simulink model "hexapod"  (R2022a)
settings: Solver=ode2  StartTime=0.0  StopTime=10.0  FixedStep=1e-4  RelTol=1e-3  AbsTol=1e-3  EnableMultiTasking=on
values from neighbouring files (symbols this model uses):
  N = 2    [gen_singleGait.m]
  s = t/T    [gait_mv_backward.m]    (also in gait_mv_forward.m; gait_mv_left.m; gait_mv_right.m; gait_rot_clockwise.m)
undefined symbols (not defined in the file or in its folder): X, Y, Z
libraries: sm_lib x90, nesl_utility x19, Contact_Forces_Lib x6, simulink x1
(part 2 of 4)

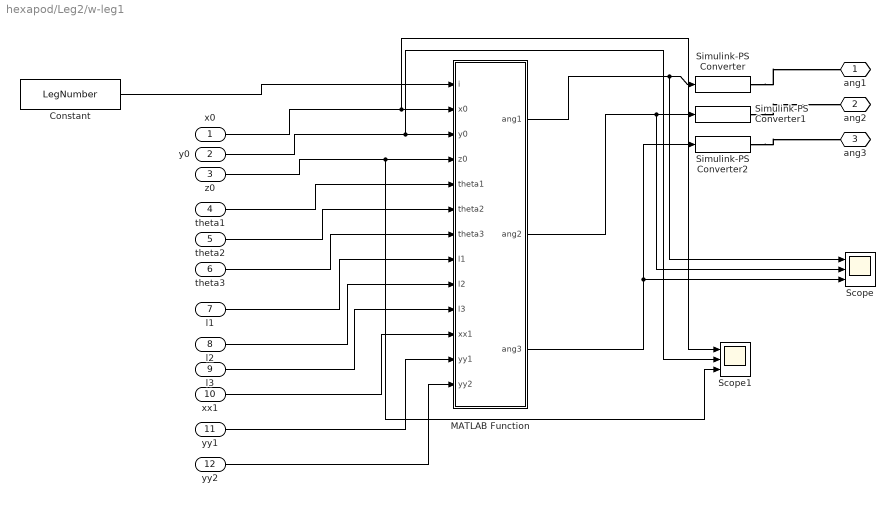
== system hexapod/Leg2/w-leg1 ==
  x0 : Inport
  y0 : Inport  Port=2
  z0 : Inport  Port=3
  theta1 : Inport  Port=4
  theta2 : Inport  Port=5
  theta3 : Inport  Port=6
  l1 : Inport  Port=7
  l2 : Inport  Port=8
  l3 : Inport  Port=9
  xx1 : Inport  Port=10
  yy1 : Inport  Port=11
  yy2 : Inport  Port=12
  Constant : Constant  Value=LegNumber
  MATLAB Function : MATLAB Function  TreatAsAtomicUnit=on
  Scope : Scope  NumInputPorts=3
  Scope1 : Scope  NumInputPorts=3
  Simulink-PS Converter : nesl_utility/Simulink-PS Converter  PhysicalDomain=network_engine_domain  SubClassName=ps_input  LeftPortType=input  RightPortType=output  PseudoPeriodic=off  Frequencies=[]  NoiseDistribution=none  NoiseParameters=[]  Unit=1  AffineConversion=off  FilteringAndDerivatives=filter  SimscapeFilterOrder=2  InputFilterTimeConstant=0.001  UdotUserProvided=0
      settings: SourceProductBaseCode=SS,PW,VE
  Simulink-PS Converter1 : nesl_utility/Simulink-PS Converter  PhysicalDomain=network_engine_domain  SubClassName=ps_input  LeftPortType=input  RightPortType=output  PseudoPeriodic=off  Frequencies=[]  NoiseDistribution=none  NoiseParameters=[]  Unit=1  AffineConversion=off  FilteringAndDerivatives=filter  SimscapeFilterOrder=2  InputFilterTimeConstant=0.001  UdotUserProvided=0
      settings: SourceProductBaseCode=SS,PW,VE
  Simulink-PS Converter2 : nesl_utility/Simulink-PS Converter  PhysicalDomain=network_engine_domain  SubClassName=ps_input  LeftPortType=input  RightPortType=output  PseudoPeriodic=off  Frequencies=[]  NoiseDistribution=none  NoiseParameters=[]  Unit=1  AffineConversion=off  FilteringAndDerivatives=filter  SimscapeFilterOrder=2  InputFilterTimeConstant=0.001  UdotUserProvided=0
      settings: SourceProductBaseCode=SS,PW,VE
  ang1 : PMIOPort  Side=Right
  ang2 : PMIOPort  Port=2  Side=Right
  ang3 : PMIOPort  Port=3  Side=Right
  wires:
  l3/1 -> MATLAB Function/10(l3)
  l2/1 -> MATLAB Function/9(l2)
  l1/1 -> MATLAB Function/8(l1)
  theta3/1 -> MATLAB Function/7(theta3)
  theta2/1 -> MATLAB Function/6(theta2)
  theta1/1 -> MATLAB Function/5(theta1)
  MATLAB Function/3(ang3) -> Simulink-PS Converter2/1, Scope/3
  MATLAB Function/2(ang2) -> Scope/2, Simulink-PS Converter1/1
  y0/1 -> Scope1/2, MATLAB Function/3(y0)
  Constant/1 -> MATLAB Function/1(i)
  MATLAB Function/1(ang1) -> Scope/1, Simulink-PS Converter/1
  z0/1 -> Scope1/3, MATLAB Function/4(z0)
  x0/1 -> Scope1/1, MATLAB Function/2(x0)
  xx1/1 -> MATLAB Function/11(xx1)
  yy1/1 -> MATLAB Function/12(yy1)
  yy2/1 -> MATLAB Function/13(yy2)
  connections:
  Simulink-PS Converter/RConn1 -- ang1/RConn1
  Simulink-PS Converter1/RConn1 -- ang2/RConn1
  Simulink-PS Converter2/RConn1 -- ang3/RConn1

== system hexapod/Leg3/leg1 ==
  Revolute Joint : sm_lib/Joints/Revolute Joint  JointMode=Normal  SenseConstraintForce=off  SenseConstraintForceX=off  SenseConstraintForceY=off  SenseConstraintForceZ=off  SenseConstraintTorque=off  SenseConstraintTorqueX=off  SenseConstraintTorqueY=off  SenseConstraintTorqueZ=off  SenseTotalForce=off  SenseTotalForceX=off  SenseTotalForceY=off  SenseTotalForceZ=off  SenseTotalTorque=off  SenseTotalTorqueX=off  SenseTotalTorqueY=off  SenseTotalTorqueZ=off  CompositeWrenchDir=FollowerOnBase  CompositeWrenchFrame=BaseFrame  EquilibriumPosition=0  EquilibriumPositionUnits=deg  SpringStiffness=0  SpringStiffnessUnits=N*m/deg  DampingCoefficient=0  DampingCoefficientUnits=N*m/(deg/s)  TorqueActuationMode=ComputedTorque  MotionActuationMode=InputMotion  SensePosition=off  SenseVelocity=off  SenseAcceleration=off  SenseTorqueForce=off  SenseLowerLimitTorqueForce=off  SenseUpperLimitTorqueForce=off  LowerLimitSpecify=off  LowerLimitBound=-90  LowerLimitBoundUnits=deg  LowerLimitStiffness=1e4  LowerLimitStiffnessUnits=N*m/deg  LowerLimitDamping=10  LowerLimitDampingUnits=N*m/(deg/s)  LowerLimitTransitionRegionWidth=0.1  LowerLimitTransitionRegionWidthUnits=deg  UpperLimitSpecify=off  UpperLimitBound=90  UpperLimitBoundUnits=deg  UpperLimitStiffness=1e4  UpperLimitStiffnessUnits=N*m/deg  UpperLimitDamping=10  UpperLimitDampingUnits=N*m/(deg/s)  UpperLimitTransitionRegionWidth=0.1  UpperLimitTransitionRegionWidthUnits=deg  PositionTargetSpecify=off  PositionTargetPriority=High  PositionTargetValue=0  PositionTargetValueUnits=deg  VelocityTargetSpecify=off  VelocityTargetPriority=High  VelocityTargetValue=0  VelocityTargetValueUnits=deg/s
  Revolute Joint1 : sm_lib/Joints/Revolute Joint  JointMode=Normal  SenseConstraintForce=off  SenseConstraintForceX=off  SenseConstraintForceY=off  SenseConstraintForceZ=off  SenseConstraintTorque=off  SenseConstraintTorqueX=off  SenseConstraintTorqueY=off  SenseConstraintTorqueZ=off  SenseTotalForce=off  SenseTotalForceX=off  SenseTotalForceY=off  SenseTotalForceZ=off  SenseTotalTorque=off  SenseTotalTorqueX=off  SenseTotalTorqueY=off  SenseTotalTorqueZ=off  CompositeWrenchDir=FollowerOnBase  CompositeWrenchFrame=BaseFrame  EquilibriumPosition=0  EquilibriumPositionUnits=deg  SpringStiffness=0  SpringStiffnessUnits=N*m/deg  DampingCoefficient=0  DampingCoefficientUnits=N*m/(deg/s)  TorqueActuationMode=ComputedTorque  MotionActuationMode=InputMotion  SensePosition=off  SenseVelocity=off  SenseAcceleration=off  SenseTorqueForce=off  SenseLowerLimitTorqueForce=off  SenseUpperLimitTorqueForce=off  LowerLimitSpecify=off  LowerLimitBound=-90  LowerLimitBoundUnits=deg  LowerLimitStiffness=1e4  LowerLimitStiffnessUnits=N*m/deg  LowerLimitDamping=10  LowerLimitDampingUnits=N*m/(deg/s)  LowerLimitTransitionRegionWidth=0.1  LowerLimitTransitionRegionWidthUnits=deg  UpperLimitSpecify=off  UpperLimitBound=90  UpperLimitBoundUnits=deg  UpperLimitStiffness=1e4  UpperLimitStiffnessUnits=N*m/deg  UpperLimitDamping=10  UpperLimitDampingUnits=N*m/(deg/s)  UpperLimitTransitionRegionWidth=0.1  UpperLimitTransitionRegionWidthUnits=deg  PositionTargetSpecify=off  PositionTargetPriority=High  PositionTargetValue=0  PositionTargetValueUnits=deg  VelocityTargetSpecify=off  VelocityTargetPriority=High  VelocityTargetValue=0  VelocityTargetValueUnits=deg/s
  Revolute Joint2 : sm_lib/Joints/Revolute Joint  JointMode=Normal  SenseConstraintForce=off  SenseConstraintForceX=off  SenseConstraintForceY=off  SenseConstraintForceZ=off  SenseConstraintTorque=off  SenseConstraintTorqueX=off  SenseConstraintTorqueY=off  SenseConstraintTorqueZ=off  SenseTotalForce=off  SenseTotalForceX=off  SenseTotalForceY=off  SenseTotalForceZ=off  SenseTotalTorque=off  SenseTotalTorqueX=off  SenseTotalTorqueY=off  SenseTotalTorqueZ=off  CompositeWrenchDir=FollowerOnBase  CompositeWrenchFrame=BaseFrame  EquilibriumPosition=0  EquilibriumPositionUnits=deg  SpringStiffness=0  SpringStiffnessUnits=N*m/deg  DampingCoefficient=0  DampingCoefficientUnits=N*m/(deg/s)  TorqueActuationMode=ComputedTorque  MotionActuationMode=InputMotion  SensePosition=off  SenseVelocity=off  SenseAcceleration=off  SenseTorqueForce=off  SenseLowerLimitTorqueForce=off  SenseUpperLimitTorqueForce=off  LowerLimitSpecify=off  LowerLimitBound=-90  LowerLimitBoundUnits=deg  LowerLimitStiffness=1e4  LowerLimitStiffnessUnits=N*m/deg  LowerLimitDamping=10  LowerLimitDampingUnits=N*m/(deg/s)  LowerLimitTransitionRegionWidth=0.1  LowerLimitTransitionRegionWidthUnits=deg  UpperLimitSpecify=off  UpperLimitBound=90  UpperLimitBoundUnits=deg  UpperLimitStiffness=1e4  UpperLimitStiffnessUnits=N*m/deg  UpperLimitDamping=10  UpperLimitDampingUnits=N*m/(deg/s)  UpperLimitTransitionRegionWidth=0.1  UpperLimitTransitionRegionWidthUnits=deg  PositionTargetSpecify=off  PositionTargetPriority=High  PositionTargetValue=0  PositionTargetValueUnits=deg  VelocityTargetSpecify=off  VelocityTargetPriority=High  VelocityTargetValue=0  VelocityTargetValueUnits=deg/s
  link1 : Subsystem
  link2 : Subsystem
  link3 : Subsystem
  base : PMIOPort  Side=Left
  ang1 : PMIOPort  Port=2  Side=Left
  ang2 : PMIOPort  Port=3  Side=Left
  ang3 : PMIOPort  Port=4  Side=Left
  end : PMIOPort  Port=5  Side=Right
  connections:
  Revolute Joint2/LConn2 -- ang3/RConn1
  Revolute Joint/LConn2 -- ang1/RConn1
  Revolute Joint/RConn1 -- link1/LConn1
  Revolute Joint2/RConn1 -- link3/LConn1
  Revolute Joint1/LConn1 -- link1/RConn1
  link2/LConn1 -- Revolute Joint1/RConn1
  Revolute Joint2/LConn1 -- link2/RConn1
  end/RConn1 -- link3/RConn1
  base/RConn1 -- Revolute Joint/LConn1
  Revolute Joint1/LConn2 -- ang2/RConn1

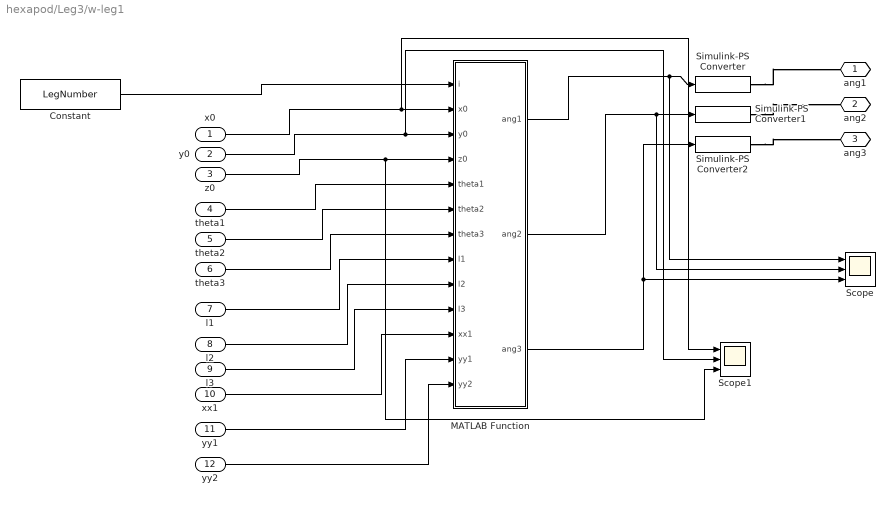
== system hexapod/Leg3/w-leg1 ==
  x0 : Inport
  y0 : Inport  Port=2
  z0 : Inport  Port=3
  theta1 : Inport  Port=4
  theta2 : Inport  Port=5
  theta3 : Inport  Port=6
  l1 : Inport  Port=7
  l2 : Inport  Port=8
  l3 : Inport  Port=9
  xx1 : Inport  Port=10
  yy1 : Inport  Port=11
  yy2 : Inport  Port=12
  Constant : Constant  Value=LegNumber
  MATLAB Function : MATLAB Function  TreatAsAtomicUnit=on
  Scope : Scope  NumInputPorts=3
  Scope1 : Scope  NumInputPorts=3
  Simulink-PS Converter : nesl_utility/Simulink-PS Converter  PhysicalDomain=network_engine_domain  SubClassName=ps_input  LeftPortType=input  RightPortType=output  PseudoPeriodic=off  Frequencies=[]  NoiseDistribution=none  NoiseParameters=[]  Unit=1  AffineConversion=off  FilteringAndDerivatives=filter  SimscapeFilterOrder=2  InputFilterTimeConstant=0.001  UdotUserProvided=0
      settings: SourceProductBaseCode=SS,PW,VE
  Simulink-PS Converter1 : nesl_utility/Simulink-PS Converter  PhysicalDomain=network_engine_domain  SubClassName=ps_input  LeftPortType=input  RightPortType=output  PseudoPeriodic=off  Frequencies=[]  NoiseDistribution=none  NoiseParameters=[]  Unit=1  AffineConversion=off  FilteringAndDerivatives=filter  SimscapeFilterOrder=2  InputFilterTimeConstant=0.001  UdotUserProvided=0
      settings: SourceProductBaseCode=SS,PW,VE
  Simulink-PS Converter2 : nesl_utility/Simulink-PS Converter  PhysicalDomain=network_engine_domain  SubClassName=ps_input  LeftPortType=input  RightPortType=output  PseudoPeriodic=off  Frequencies=[]  NoiseDistribution=none  NoiseParameters=[]  Unit=1  AffineConversion=off  FilteringAndDerivatives=filter  SimscapeFilterOrder=2  InputFilterTimeConstant=0.001  UdotUserProvided=0
      settings: SourceProductBaseCode=SS,PW,VE
  ang1 : PMIOPort  Side=Right
  ang2 : PMIOPort  Port=2  Side=Right
  ang3 : PMIOPort  Port=3  Side=Right
  wires:
  yy2/1 -> MATLAB Function/13(yy2)
  yy1/1 -> MATLAB Function/12(yy1)
  xx1/1 -> MATLAB Function/11(xx1)
  x0/1 -> MATLAB Function/2(x0), Scope1/1
  z0/1 -> MATLAB Function/4(z0), Scope1/3
  MATLAB Function/1(ang1) -> Simulink-PS Converter/1, Scope/1
  Constant/1 -> MATLAB Function/1(i)
  y0/1 -> MATLAB Function/3(y0), Scope1/2
  MATLAB Function/2(ang2) -> Simulink-PS Converter1/1, Scope/2
  MATLAB Function/3(ang3) -> Scope/3, Simulink-PS Converter2/1
  theta1/1 -> MATLAB Function/5(theta1)
  theta2/1 -> MATLAB Function/6(theta2)
  theta3/1 -> MATLAB Function/7(theta3)
  l1/1 -> MATLAB Function/8(l1)
  l2/1 -> MATLAB Function/9(l2)
  l3/1 -> MATLAB Function/10(l3)
  connections:
  Simulink-PS Converter2/RConn1 -- ang3/RConn1
  Simulink-PS Converter1/RConn1 -- ang2/RConn1
  Simulink-PS Converter/RConn1 -- ang1/RConn1

== system hexapod/Leg4/leg1 ==
  Revolute Joint : sm_lib/Joints/Revolute Joint  JointMode=Normal  SenseConstraintForce=off  SenseConstraintForceX=off  SenseConstraintForceY=off  SenseConstraintForceZ=off  SenseConstraintTorque=off  SenseConstraintTorqueX=off  SenseConstraintTorqueY=off  SenseConstraintTorqueZ=off  SenseTotalForce=off  SenseTotalForceX=off  SenseTotalForceY=off  SenseTotalForceZ=off  SenseTotalTorque=off  SenseTotalTorqueX=off  SenseTotalTorqueY=off  SenseTotalTorqueZ=off  CompositeWrenchDir=FollowerOnBase  CompositeWrenchFrame=BaseFrame  EquilibriumPosition=0  EquilibriumPositionUnits=deg  SpringStiffness=0  SpringStiffnessUnits=N*m/deg  DampingCoefficient=0  DampingCoefficientUnits=N*m/(deg/s)  TorqueActuationMode=ComputedTorque  MotionActuationMode=InputMotion  SensePosition=off  SenseVelocity=off  SenseAcceleration=off  SenseTorqueForce=off  SenseLowerLimitTorqueForce=off  SenseUpperLimitTorqueForce=off  LowerLimitSpecify=off  LowerLimitBound=-90  LowerLimitBoundUnits=deg  LowerLimitStiffness=1e4  LowerLimitStiffnessUnits=N*m/deg  LowerLimitDamping=10  LowerLimitDampingUnits=N*m/(deg/s)  LowerLimitTransitionRegionWidth=0.1  LowerLimitTransitionRegionWidthUnits=deg  UpperLimitSpecify=off  UpperLimitBound=90  UpperLimitBoundUnits=deg  UpperLimitStiffness=1e4  UpperLimitStiffnessUnits=N*m/deg  UpperLimitDamping=10  UpperLimitDampingUnits=N*m/(deg/s)  UpperLimitTransitionRegionWidth=0.1  UpperLimitTransitionRegionWidthUnits=deg  PositionTargetSpecify=off  PositionTargetPriority=High  PositionTargetValue=0  PositionTargetValueUnits=deg  VelocityTargetSpecify=off  VelocityTargetPriority=High  VelocityTargetValue=0  VelocityTargetValueUnits=deg/s
  Revolute Joint1 : sm_lib/Joints/Revolute Joint  JointMode=Normal  SenseConstraintForce=off  SenseConstraintForceX=off  SenseConstraintForceY=off  SenseConstraintForceZ=off  SenseConstraintTorque=off  SenseConstraintTorqueX=off  SenseConstraintTorqueY=off  SenseConstraintTorqueZ=off  SenseTotalForce=off  SenseTotalForceX=off  SenseTotalForceY=off  SenseTotalForceZ=off  SenseTotalTorque=off  SenseTotalTorqueX=off  SenseTotalTorqueY=off  SenseTotalTorqueZ=off  CompositeWrenchDir=FollowerOnBase  CompositeWrenchFrame=BaseFrame  EquilibriumPosition=0  EquilibriumPositionUnits=deg  SpringStiffness=0  SpringStiffnessUnits=N*m/deg  DampingCoefficient=0  DampingCoefficientUnits=N*m/(deg/s)  TorqueActuationMode=ComputedTorque  MotionActuationMode=InputMotion  SensePosition=off  SenseVelocity=off  SenseAcceleration=off  SenseTorqueForce=off  SenseLowerLimitTorqueForce=off  SenseUpperLimitTorqueForce=off  LowerLimitSpecify=off  LowerLimitBound=-90  LowerLimitBoundUnits=deg  LowerLimitStiffness=1e4  LowerLimitStiffnessUnits=N*m/deg  LowerLimitDamping=10  LowerLimitDampingUnits=N*m/(deg/s)  LowerLimitTransitionRegionWidth=0.1  LowerLimitTransitionRegionWidthUnits=deg  UpperLimitSpecify=off  UpperLimitBound=90  UpperLimitBoundUnits=deg  UpperLimitStiffness=1e4  UpperLimitStiffnessUnits=N*m/deg  UpperLimitDamping=10  UpperLimitDampingUnits=N*m/(deg/s)  UpperLimitTransitionRegionWidth=0.1  UpperLimitTransitionRegionWidthUnits=deg  PositionTargetSpecify=off  PositionTargetPriority=High  PositionTargetValue=0  PositionTargetValueUnits=deg  VelocityTargetSpecify=off  VelocityTargetPriority=High  VelocityTargetValue=0  VelocityTargetValueUnits=deg/s
  Revolute Joint2 : sm_lib/Joints/Revolute Joint  JointMode=Normal  SenseConstraintForce=off  SenseConstraintForceX=off  SenseConstraintForceY=off  SenseConstraintForceZ=off  SenseConstraintTorque=off  SenseConstraintTorqueX=off  SenseConstraintTorqueY=off  SenseConstraintTorqueZ=off  SenseTotalForce=off  SenseTotalForceX=off  SenseTotalForceY=off  SenseTotalForceZ=off  SenseTotalTorque=off  SenseTotalTorqueX=off  SenseTotalTorqueY=off  SenseTotalTorqueZ=off  CompositeWrenchDir=FollowerOnBase  CompositeWrenchFrame=BaseFrame  EquilibriumPosition=0  EquilibriumPositionUnits=deg  SpringStiffness=0  SpringStiffnessUnits=N*m/deg  DampingCoefficient=0  DampingCoefficientUnits=N*m/(deg/s)  TorqueActuationMode=ComputedTorque  MotionActuationMode=InputMotion  SensePosition=off  SenseVelocity=off  SenseAcceleration=off  SenseTorqueForce=off  SenseLowerLimitTorqueForce=off  SenseUpperLimitTorqueForce=off  LowerLimitSpecify=off  LowerLimitBound=-90  LowerLimitBoundUnits=deg  LowerLimitStiffness=1e4  LowerLimitStiffnessUnits=N*m/deg  LowerLimitDamping=10  LowerLimitDampingUnits=N*m/(deg/s)  LowerLimitTransitionRegionWidth=0.1  LowerLimitTransitionRegionWidthUnits=deg  UpperLimitSpecify=off  UpperLimitBound=90  UpperLimitBoundUnits=deg  UpperLimitStiffness=1e4  UpperLimitStiffnessUnits=N*m/deg  UpperLimitDamping=10  UpperLimitDampingUnits=N*m/(deg/s)  UpperLimitTransitionRegionWidth=0.1  UpperLimitTransitionRegionWidthUnits=deg  PositionTargetSpecify=off  PositionTargetPriority=High  PositionTargetValue=0  PositionTargetValueUnits=deg  VelocityTargetSpecify=off  VelocityTargetPriority=High  VelocityTargetValue=0  VelocityTargetValueUnits=deg/s
  link1 : Subsystem
  link2 : Subsystem
  link3 : Subsystem
  base : PMIOPort  Side=Left
  ang1 : PMIOPort  Port=2  Side=Left
  ang2 : PMIOPort  Port=3  Side=Left
  ang3 : PMIOPort  Port=4  Side=Left
  end : PMIOPort  Port=5  Side=Right
  connections:
  Revolute Joint1/LConn2 -- ang2/RConn1
  base/RConn1 -- Revolute Joint/LConn1
  end/RConn1 -- link3/RConn1
  Revolute Joint2/LConn1 -- link2/RConn1
  link2/LConn1 -- Revolute Joint1/RConn1
  Revolute Joint1/LConn1 -- link1/RConn1
  Revolute Joint2/RConn1 -- link3/LConn1
  Revolute Joint/RConn1 -- link1/LConn1
  Revolute Joint/LConn2 -- ang1/RConn1
  Revolute Joint2/LConn2 -- ang3/RConn1

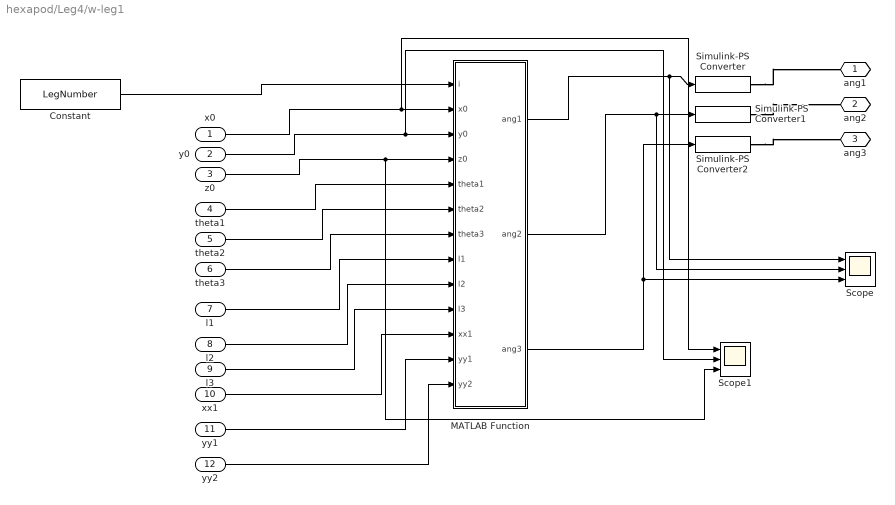
== system hexapod/Leg4/w-leg1 ==
  x0 : Inport
  y0 : Inport  Port=2
  z0 : Inport  Port=3
  theta1 : Inport  Port=4
  theta2 : Inport  Port=5
  theta3 : Inport  Port=6
  l1 : Inport  Port=7
  l2 : Inport  Port=8
  l3 : Inport  Port=9
  xx1 : Inport  Port=10
  yy1 : Inport  Port=11
  yy2 : Inport  Port=12
  Constant : Constant  Value=LegNumber
  MATLAB Function : MATLAB Function  TreatAsAtomicUnit=on
  Scope : Scope  NumInputPorts=3
  Scope1 : Scope  NumInputPorts=3
  Simulink-PS Converter : nesl_utility/Simulink-PS Converter  PhysicalDomain=network_engine_domain  SubClassName=ps_input  LeftPortType=input  RightPortType=output  PseudoPeriodic=off  Frequencies=[]  NoiseDistribution=none  NoiseParameters=[]  Unit=1  AffineConversion=off  FilteringAndDerivatives=filter  SimscapeFilterOrder=2  InputFilterTimeConstant=0.001  UdotUserProvided=0
      settings: SourceProductBaseCode=SS,PW,VE
  Simulink-PS Converter1 : nesl_utility/Simulink-PS Converter  PhysicalDomain=network_engine_domain  SubClassName=ps_input  LeftPortType=input  RightPortType=output  PseudoPeriodic=off  Frequencies=[]  NoiseDistribution=none  NoiseParameters=[]  Unit=1  AffineConversion=off  FilteringAndDerivatives=filter  SimscapeFilterOrder=2  InputFilterTimeConstant=0.001  UdotUserProvided=0
      settings: SourceProductBaseCode=SS,PW,VE
  Simulink-PS Converter2 : nesl_utility/Simulink-PS Converter  PhysicalDomain=network_engine_domain  SubClassName=ps_input  LeftPortType=input  RightPortType=output  PseudoPeriodic=off  Frequencies=[]  NoiseDistribution=none  NoiseParameters=[]  Unit=1  AffineConversion=off  FilteringAndDerivatives=filter  SimscapeFilterOrder=2  InputFilterTimeConstant=0.001  UdotUserProvided=0
      settings: SourceProductBaseCode=SS,PW,VE
  ang1 : PMIOPort  Side=Right
  ang2 : PMIOPort  Port=2  Side=Right
  ang3 : PMIOPort  Port=3  Side=Right
  wires:
  l3/1 -> MATLAB Function/10(l3)
  l2/1 -> MATLAB Function/9(l2)
  l1/1 -> MATLAB Function/8(l1)
  theta3/1 -> MATLAB Function/7(theta3)
  theta2/1 -> MATLAB Function/6(theta2)
  theta1/1 -> MATLAB Function/5(theta1)
  MATLAB Function/3(ang3) -> Simulink-PS Converter2/1, Scope/3
  MATLAB Function/2(ang2) -> Scope/2, Simulink-PS Converter1/1
  y0/1 -> Scope1/2, MATLAB Function/3(y0)
  Constant/1 -> MATLAB Function/1(i)
  MATLAB Function/1(ang1) -> Scope/1, Simulink-PS Converter/1
  z0/1 -> Scope1/3, MATLAB Function/4(z0)
  x0/1 -> Scope1/1, MATLAB Function/2(x0)
  xx1/1 -> MATLAB Function/11(xx1)
  yy1/1 -> MATLAB Function/12(yy1)
  yy2/1 -> MATLAB Function/13(yy2)
  connections:
  Simulink-PS Converter/RConn1 -- ang1/RConn1
  Simulink-PS Converter1/RConn1 -- ang2/RConn1
  Simulink-PS Converter2/RConn1 -- ang3/RConn1

== system hexapod/Leg5/leg1 ==
  Revolute Joint : sm_lib/Joints/Revolute Joint  JointMode=Normal  SenseConstraintForce=off  SenseConstraintForceX=off  SenseConstraintForceY=off  SenseConstraintForceZ=off  SenseConstraintTorque=off  SenseConstraintTorqueX=off  SenseConstraintTorqueY=off  SenseConstraintTorqueZ=off  SenseTotalForce=off  SenseTotalForceX=off  SenseTotalForceY=off  SenseTotalForceZ=off  SenseTotalTorque=off  SenseTotalTorqueX=off  SenseTotalTorqueY=off  SenseTotalTorqueZ=off  CompositeWrenchDir=FollowerOnBase  CompositeWrenchFrame=BaseFrame  EquilibriumPosition=0  EquilibriumPositionUnits=deg  SpringStiffness=0  SpringStiffnessUnits=N*m/deg  DampingCoefficient=0  DampingCoefficientUnits=N*m/(deg/s)  TorqueActuationMode=ComputedTorque  MotionActuationMode=InputMotion  SensePosition=off  SenseVelocity=off  SenseAcceleration=off  SenseTorqueForce=off  SenseLowerLimitTorqueForce=off  SenseUpperLimitTorqueForce=off  LowerLimitSpecify=off  LowerLimitBound=-90  LowerLimitBoundUnits=deg  LowerLimitStiffness=1e4  LowerLimitStiffnessUnits=N*m/deg  LowerLimitDamping=10  LowerLimitDampingUnits=N*m/(deg/s)  LowerLimitTransitionRegionWidth=0.1  LowerLimitTransitionRegionWidthUnits=deg  UpperLimitSpecify=off  UpperLimitBound=90  UpperLimitBoundUnits=deg  UpperLimitStiffness=1e4  UpperLimitStiffnessUnits=N*m/deg  UpperLimitDamping=10  UpperLimitDampingUnits=N*m/(deg/s)  UpperLimitTransitionRegionWidth=0.1  UpperLimitTransitionRegionWidthUnits=deg  PositionTargetSpecify=off  PositionTargetPriority=High  PositionTargetValue=0  PositionTargetValueUnits=deg  VelocityTargetSpecify=off  VelocityTargetPriority=High  VelocityTargetValue=0  VelocityTargetValueUnits=deg/s
  Revolute Joint1 : sm_lib/Joints/Revolute Joint  JointMode=Normal  SenseConstraintForce=off  SenseConstraintForceX=off  SenseConstraintForceY=off  SenseConstraintForceZ=off  SenseConstraintTorque=off  SenseConstraintTorqueX=off  SenseConstraintTorqueY=off  SenseConstraintTorqueZ=off  SenseTotalForce=off  SenseTotalForceX=off  SenseTotalForceY=off  SenseTotalForceZ=off  SenseTotalTorque=off  SenseTotalTorqueX=off  SenseTotalTorqueY=off  SenseTotalTorqueZ=off  CompositeWrenchDir=FollowerOnBase  CompositeWrenchFrame=BaseFrame  EquilibriumPosition=0  EquilibriumPositionUnits=deg  SpringStiffness=0  SpringStiffnessUnits=N*m/deg  DampingCoefficient=0  DampingCoefficientUnits=N*m/(deg/s)  TorqueActuationMode=ComputedTorque  MotionActuationMode=InputMotion  SensePosition=off  SenseVelocity=off  SenseAcceleration=off  SenseTorqueForce=off  SenseLowerLimitTorqueForce=off  SenseUpperLimitTorqueForce=off  LowerLimitSpecify=off  LowerLimitBound=-90  LowerLimitBoundUnits=deg  LowerLimitStiffness=1e4  LowerLimitStiffnessUnits=N*m/deg  LowerLimitDamping=10  LowerLimitDampingUnits=N*m/(deg/s)  LowerLimitTransitionRegionWidth=0.1  LowerLimitTransitionRegionWidthUnits=deg  UpperLimitSpecify=off  UpperLimitBound=90  UpperLimitBoundUnits=deg  UpperLimitStiffness=1e4  UpperLimitStiffnessUnits=N*m/deg  UpperLimitDamping=10  UpperLimitDampingUnits=N*m/(deg/s)  UpperLimitTransitionRegionWidth=0.1  UpperLimitTransitionRegionWidthUnits=deg  PositionTargetSpecify=off  PositionTargetPriority=High  PositionTargetValue=0  PositionTargetValueUnits=deg  VelocityTargetSpecify=off  VelocityTargetPriority=High  VelocityTargetValue=0  VelocityTargetValueUnits=deg/s
  Revolute Joint2 : sm_lib/Joints/Revolute Joint  JointMode=Normal  SenseConstraintForce=off  SenseConstraintForceX=off  SenseConstraintForceY=off  SenseConstraintForceZ=off  SenseConstraintTorque=off  SenseConstraintTorqueX=off  SenseConstraintTorqueY=off  SenseConstraintTorqueZ=off  SenseTotalForce=off  SenseTotalForceX=off  SenseTotalForceY=off  SenseTotalForceZ=off  SenseTotalTorque=off  SenseTotalTorqueX=off  SenseTotalTorqueY=off  SenseTotalTorqueZ=off  CompositeWrenchDir=FollowerOnBase  CompositeWrenchFrame=BaseFrame  EquilibriumPosition=0  EquilibriumPositionUnits=deg  SpringStiffness=0  SpringStiffnessUnits=N*m/deg  DampingCoefficient=0  DampingCoefficientUnits=N*m/(deg/s)  TorqueActuationMode=ComputedTorque  MotionActuationMode=InputMotion  SensePosition=off  SenseVelocity=off  SenseAcceleration=off  SenseTorqueForce=off  SenseLowerLimitTorqueForce=off  SenseUpperLimitTorqueForce=off  LowerLimitSpecify=off  LowerLimitBound=-90  LowerLimitBoundUnits=deg  LowerLimitStiffness=1e4  LowerLimitStiffnessUnits=N*m/deg  LowerLimitDamping=10  LowerLimitDampingUnits=N*m/(deg/s)  LowerLimitTransitionRegionWidth=0.1  LowerLimitTransitionRegionWidthUnits=deg  UpperLimitSpecify=off  UpperLimitBound=90  UpperLimitBoundUnits=deg  UpperLimitStiffness=1e4  UpperLimitStiffnessUnits=N*m/deg  UpperLimitDamping=10  UpperLimitDampingUnits=N*m/(deg/s)  UpperLimitTransitionRegionWidth=0.1  UpperLimitTransitionRegionWidthUnits=deg  PositionTargetSpecify=off  PositionTargetPriority=High  PositionTargetValue=0  PositionTargetValueUnits=deg  VelocityTargetSpecify=off  VelocityTargetPriority=High  VelocityTargetValue=0  VelocityTargetValueUnits=deg/s
  link1 : Subsystem
  link2 : Subsystem
  link3 : Subsystem
  base : PMIOPort  Side=Left
  ang1 : PMIOPort  Port=2  Side=Left
  ang2 : PMIOPort  Port=3  Side=Left
  ang3 : PMIOPort  Port=4  Side=Left
  end : PMIOPort  Port=5  Side=Right
  connections:
  Revolute Joint2/LConn2 -- ang3/RConn1
  Revolute Joint/LConn2 -- ang1/RConn1
  Revolute Joint/RConn1 -- link1/LConn1
  Revolute Joint2/RConn1 -- link3/LConn1
  Revolute Joint1/LConn1 -- link1/RConn1
  link2/LConn1 -- Revolute Joint1/RConn1
  Revolute Joint2/LConn1 -- link2/RConn1
  end/RConn1 -- link3/RConn1
  base/RConn1 -- Revolute Joint/LConn1
  Revolute Joint1/LConn2 -- ang2/RConn1

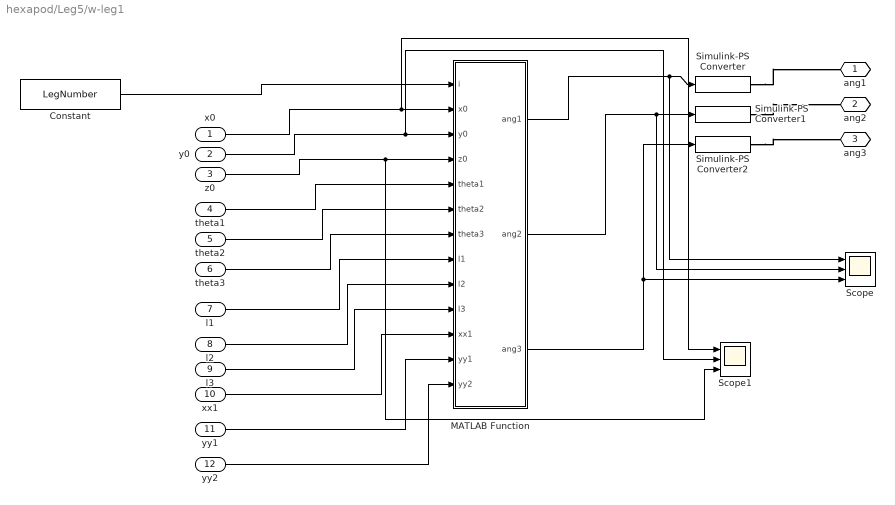
== system hexapod/Leg5/w-leg1 ==
  x0 : Inport
  y0 : Inport  Port=2
  z0 : Inport  Port=3
  theta1 : Inport  Port=4
  theta2 : Inport  Port=5
  theta3 : Inport  Port=6
  l1 : Inport  Port=7
  l2 : Inport  Port=8
  l3 : Inport  Port=9
  xx1 : Inport  Port=10
  yy1 : Inport  Port=11
  yy2 : Inport  Port=12
  Constant : Constant  Value=LegNumber
  MATLAB Function : MATLAB Function  TreatAsAtomicUnit=on
  Scope : Scope  NumInputPorts=3
  Scope1 : Scope  NumInputPorts=3
  Simulink-PS Converter : nesl_utility/Simulink-PS Converter  PhysicalDomain=network_engine_domain  SubClassName=ps_input  LeftPortType=input  RightPortType=output  PseudoPeriodic=off  Frequencies=[]  NoiseDistribution=none  NoiseParameters=[]  Unit=1  AffineConversion=off  FilteringAndDerivatives=filter  SimscapeFilterOrder=2  InputFilterTimeConstant=0.001  UdotUserProvided=0
      settings: SourceProductBaseCode=SS,PW,VE
  Simulink-PS Converter1 : nesl_utility/Simulink-PS Converter  PhysicalDomain=network_engine_domain  SubClassName=ps_input  LeftPortType=input  RightPortType=output  PseudoPeriodic=off  Frequencies=[]  NoiseDistribution=none  NoiseParameters=[]  Unit=1  AffineConversion=off  FilteringAndDerivatives=filter  SimscapeFilterOrder=2  InputFilterTimeConstant=0.001  UdotUserProvided=0
      settings: SourceProductBaseCode=SS,PW,VE
  Simulink-PS Converter2 : nesl_utility/Simulink-PS Converter  PhysicalDomain=network_engine_domain  SubClassName=ps_input  LeftPortType=input  RightPortType=output  PseudoPeriodic=off  Frequencies=[]  NoiseDistribution=none  NoiseParameters=[]  Unit=1  AffineConversion=off  FilteringAndDerivatives=filter  SimscapeFilterOrder=2  InputFilterTimeConstant=0.001  UdotUserProvided=0
      settings: SourceProductBaseCode=SS,PW,VE
  ang1 : PMIOPort  Side=Right
  ang2 : PMIOPort  Port=2  Side=Right
  ang3 : PMIOPort  Port=3  Side=Right
  wires:
  yy2/1 -> MATLAB Function/13(yy2)
  yy1/1 -> MATLAB Function/12(yy1)
  xx1/1 -> MATLAB Function/11(xx1)
  x0/1 -> MATLAB Function/2(x0), Scope1/1
  z0/1 -> MATLAB Function/4(z0), Scope1/3
  MATLAB Function/1(ang1) -> Simulink-PS Converter/1, Scope/1
  Constant/1 -> MATLAB Function/1(i)
  y0/1 -> MATLAB Function/3(y0), Scope1/2
  MATLAB Function/2(ang2) -> Simulink-PS Converter1/1, Scope/2
  MATLAB Function/3(ang3) -> Scope/3, Simulink-PS Converter2/1
  theta1/1 -> MATLAB Function/5(theta1)
  theta2/1 -> MATLAB Function/6(theta2)
  theta3/1 -> MATLAB Function/7(theta3)
  l1/1 -> MATLAB Function/8(l1)
  l2/1 -> MATLAB Function/9(l2)
  l3/1 -> MATLAB Function/10(l3)
  connections:
  Simulink-PS Converter2/RConn1 -- ang3/RConn1
  Simulink-PS Converter1/RConn1 -- ang2/RConn1
  Simulink-PS Converter/RConn1 -- ang1/RConn1

== system hexapod/Leg6/leg1 ==
  Revolute Joint : sm_lib/Joints/Revolute Joint  JointMode=Normal  SenseConstraintForce=off  SenseConstraintForceX=off  SenseConstraintForceY=off  SenseConstraintForceZ=off  SenseConstraintTorque=off  SenseConstraintTorqueX=off  SenseConstraintTorqueY=off  SenseConstraintTorqueZ=off  SenseTotalForce=off  SenseTotalForceX=off  SenseTotalForceY=off  SenseTotalForceZ=off  SenseTotalTorque=off  SenseTotalTorqueX=off  SenseTotalTorqueY=off  SenseTotalTorqueZ=off  CompositeWrenchDir=FollowerOnBase  CompositeWrenchFrame=BaseFrame  EquilibriumPosition=0  EquilibriumPositionUnits=deg  SpringStiffness=0  SpringStiffnessUnits=N*m/deg  DampingCoefficient=0  DampingCoefficientUnits=N*m/(deg/s)  TorqueActuationMode=ComputedTorque  MotionActuationMode=InputMotion  SensePosition=off  SenseVelocity=off  SenseAcceleration=off  SenseTorqueForce=off  SenseLowerLimitTorqueForce=off  SenseUpperLimitTorqueForce=off  LowerLimitSpecify=off  LowerLimitBound=-90  LowerLimitBoundUnits=deg  LowerLimitStiffness=1e4  LowerLimitStiffnessUnits=N*m/deg  LowerLimitDamping=10  LowerLimitDampingUnits=N*m/(deg/s)  LowerLimitTransitionRegionWidth=0.1  LowerLimitTransitionRegionWidthUnits=deg  UpperLimitSpecify=off  UpperLimitBound=90  UpperLimitBoundUnits=deg  UpperLimitStiffness=1e4  UpperLimitStiffnessUnits=N*m/deg  UpperLimitDamping=10  UpperLimitDampingUnits=N*m/(deg/s)  UpperLimitTransitionRegionWidth=0.1  UpperLimitTransitionRegionWidthUnits=deg  PositionTargetSpecify=off  PositionTargetPriority=High  PositionTargetValue=0  PositionTargetValueUnits=deg  VelocityTargetSpecify=off  VelocityTargetPriority=High  VelocityTargetValue=0  VelocityTargetValueUnits=deg/s
  Revolute Joint1 : sm_lib/Joints/Revolute Joint  JointMode=Normal  SenseConstraintForce=off  SenseConstraintForceX=off  SenseConstraintForceY=off  SenseConstraintForceZ=off  SenseConstraintTorque=off  SenseConstraintTorqueX=off  SenseConstraintTorqueY=off  SenseConstraintTorqueZ=off  SenseTotalForce=off  SenseTotalForceX=off  SenseTotalForceY=off  SenseTotalForceZ=off  SenseTotalTorque=off  SenseTotalTorqueX=off  SenseTotalTorqueY=off  SenseTotalTorqueZ=off  CompositeWrenchDir=FollowerOnBase  CompositeWrenchFrame=BaseFrame  EquilibriumPosition=0  EquilibriumPositionUnits=deg  SpringStiffness=0  SpringStiffnessUnits=N*m/deg  DampingCoefficient=0  DampingCoefficientUnits=N*m/(deg/s)  TorqueActuationMode=ComputedTorque  MotionActuationMode=InputMotion  SensePosition=off  SenseVelocity=off  SenseAcceleration=off  SenseTorqueForce=off  SenseLowerLimitTorqueForce=off  SenseUpperLimitTorqueForce=off  LowerLimitSpecify=off  LowerLimitBound=-90  LowerLimitBoundUnits=deg  LowerLimitStiffness=1e4  LowerLimitStiffnessUnits=N*m/deg  LowerLimitDamping=10  LowerLimitDampingUnits=N*m/(deg/s)  LowerLimitTransitionRegionWidth=0.1  LowerLimitTransitionRegionWidthUnits=deg  UpperLimitSpecify=off  UpperLimitBound=90  UpperLimitBoundUnits=deg  UpperLimitStiffness=1e4  UpperLimitStiffnessUnits=N*m/deg  UpperLimitDamping=10  UpperLimitDampingUnits=N*m/(deg/s)  UpperLimitTransitionRegionWidth=0.1  UpperLimitTransitionRegionWidthUnits=deg  PositionTargetSpecify=off  PositionTargetPriority=High  PositionTargetValue=0  PositionTargetValueUnits=deg  VelocityTargetSpecify=off  VelocityTargetPriority=High  VelocityTargetValue=0  VelocityTargetValueUnits=deg/s
  Revolute Joint2 : sm_lib/Joints/Revolute Joint  JointMode=Normal  SenseConstraintForce=off  SenseConstraintForceX=off  SenseConstraintForceY=off  SenseConstraintForceZ=off  SenseConstraintTorque=off  SenseConstraintTorqueX=off  SenseConstraintTorqueY=off  SenseConstraintTorqueZ=off  SenseTotalForce=off  SenseTotalForceX=off  SenseTotalForceY=off  SenseTotalForceZ=off  SenseTotalTorque=off  SenseTotalTorqueX=off  SenseTotalTorqueY=off  SenseTotalTorqueZ=off  CompositeWrenchDir=FollowerOnBase  CompositeWrenchFrame=BaseFrame  EquilibriumPosition=0  EquilibriumPositionUnits=deg  SpringStiffness=0  SpringStiffnessUnits=N*m/deg  DampingCoefficient=0  DampingCoefficientUnits=N*m/(deg/s)  TorqueActuationMode=ComputedTorque  MotionActuationMode=InputMotion  SensePosition=off  SenseVelocity=off  SenseAcceleration=off  SenseTorqueForce=off  SenseLowerLimitTorqueForce=off  SenseUpperLimitTorqueForce=off  LowerLimitSpecify=off  LowerLimitBound=-90  LowerLimitBoundUnits=deg  LowerLimitStiffness=1e4  LowerLimitStiffnessUnits=N*m/deg  LowerLimitDamping=10  LowerLimitDampingUnits=N*m/(deg/s)  LowerLimitTransitionRegionWidth=0.1  LowerLimitTransitionRegionWidthUnits=deg  UpperLimitSpecify=off  UpperLimitBound=90  UpperLimitBoundUnits=deg  UpperLimitStiffness=1e4  UpperLimitStiffnessUnits=N*m/deg  UpperLimitDamping=10  UpperLimitDampingUnits=N*m/(deg/s)  UpperLimitTransitionRegionWidth=0.1  UpperLimitTransitionRegionWidthUnits=deg  PositionTargetSpecify=off  PositionTargetPriority=High  PositionTargetValue=0  PositionTargetValueUnits=deg  VelocityTargetSpecify=off  VelocityTargetPriority=High  VelocityTargetValue=0  VelocityTargetValueUnits=deg/s
  link1 : Subsystem
  link2 : Subsystem
  link3 : Subsystem
  base : PMIOPort  Side=Left
  ang1 : PMIOPort  Port=2  Side=Left
  ang2 : PMIOPort  Port=3  Side=Left
  ang3 : PMIOPort  Port=4  Side=Left
  end : PMIOPort  Port=5  Side=Right
  connections:
  Revolute Joint1/LConn2 -- ang2/RConn1
  base/RConn1 -- Revolute Joint/LConn1
  end/RConn1 -- link3/RConn1
  Revolute Joint2/LConn1 -- link2/RConn1
  link2/LConn1 -- Revolute Joint1/RConn1
  Revolute Joint1/LConn1 -- link1/RConn1
  Revolute Joint2/RConn1 -- link3/LConn1
  Revolute Joint/RConn1 -- link1/LConn1
  Revolute Joint/LConn2 -- ang1/RConn1
  Revolute Joint2/LConn2 -- ang3/RConn1

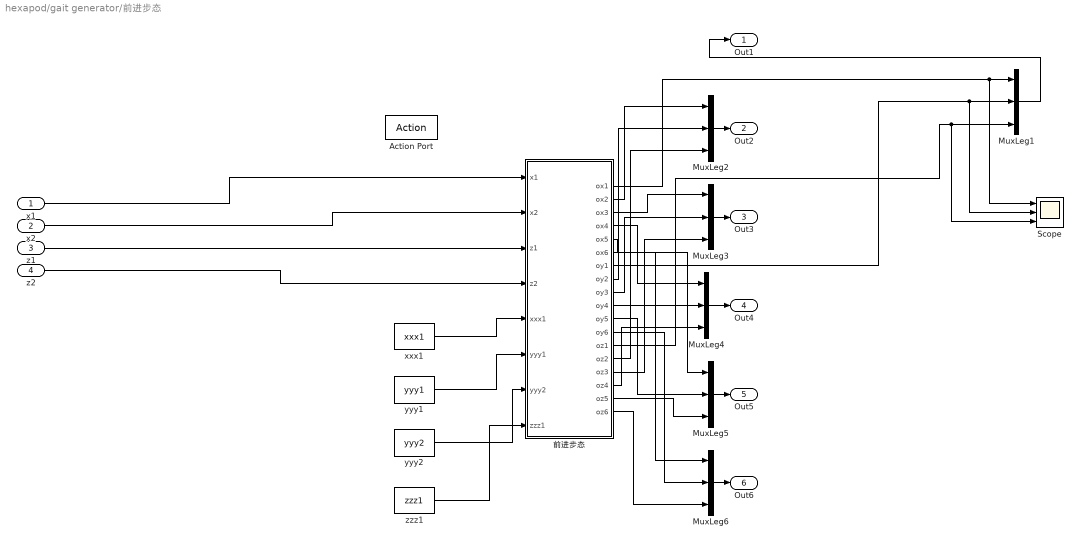
== system hexapod/gait generator/前进步态 ==
  x1 : Inport
  x2 : Inport  Port=2
  z1 : Inport  Port=3
  z2 : Inport  Port=4
  Action Port : ActionPort  ActionPortLabel=if(u1 == 1)
  MuxLeg{1..6} (6 alike) : Mux  Inputs=3
  Scope : Scope  NumInputPorts=3
  xxx1 : Constant  Value=xxx1
  yyy1 : Constant  Value=yyy1
  yyy2 : Constant  Value=yyy2
  zzz1 : Constant  Value=zzz1
  前进步态 : MATLAB Function  TreatAsAtomicUnit=on
  Out1 : Outport
  Out2 : Outport  Port=2
  Out3 : Outport  Port=3
  Out4 : Outport  Port=4
  Out5 : Outport  Port=5
  Out6 : Outport  Port=6
  wires:
  MuxLeg5/1 -> Out5/1
  MuxLeg3/1 -> Out3/1
  MuxLeg2/1 -> Out2/1
  前进步态/1(ox1) -> MuxLeg1/1, Scope/1
  前进步态/6(ox6) -> MuxLeg6/1
  前进步态/12(oy6) -> MuxLeg6/2
  z1/1 -> 前进步态/3(z1)
  前进步态/11(oy5) -> MuxLeg5/2
  z2/1 -> 前进步态/4(z2)
  前进步态/8(oy2) -> MuxLeg2/2
  前进步态/15(oz3) -> MuxLeg3/3
  前进步态/9(oy3) -> MuxLeg3/2
  前进步态/14(oz2) -> MuxLeg2/3
  前进步态/4(ox4) -> MuxLeg4/1
  MuxLeg6/1 -> Out6/1
  前进步态/10(oy4) -> MuxLeg4/2
  前进步态/5(ox5) -> MuxLeg5/1
  前进步态/2(ox2) -> MuxLeg2/1
  前进步态/16(oz4) -> MuxLeg4/3
  yyy2/1 -> 前进步态/7(yyy2)
  MuxLeg4/1 -> Out4/1
  前进步态/13(oz1) -> MuxLeg1/3, Scope/3
  前进步态/18(oz6) -> MuxLeg6/3
  zzz1/1 -> 前进步态/8(zzz1)
  MuxLeg1/1 -> Out1/1
  前进步态/3(ox3) -> MuxLeg3/1
  yyy1/1 -> 前进步态/6(yyy1)
  x2/1 -> 前进步态/2(x2)
  x1/1 -> 前进步态/1(x1)
  前进步态/7(oy1) -> MuxLeg1/2, Scope/2
  前进步态/17(oz5) -> MuxLeg5/3
  xxx1/1 -> 前进步态/5(xxx1)

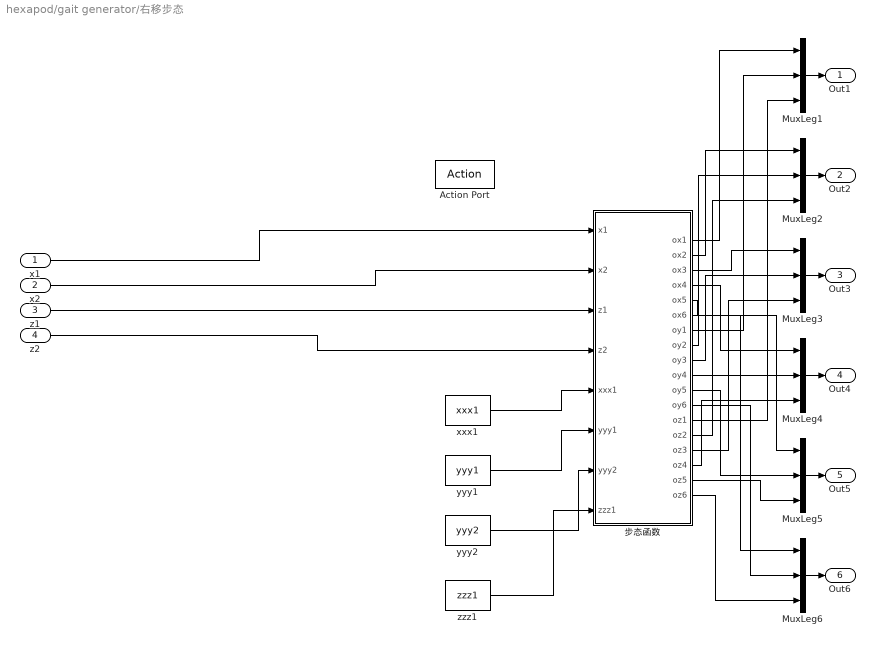
== system hexapod/gait generator/右移步态 ==
  x1 : Inport
  x2 : Inport  Port=2
  z1 : Inport  Port=3
  z2 : Inport  Port=4
  Action Port : ActionPort  ActionPortLabel=elseif(u1==4)
  MuxLeg{1..6} (6 alike) : Mux  Inputs=3
  xxx1 : Constant  Value=xxx1
  yyy1 : Constant  Value=yyy1
  yyy2 : Constant  Value=yyy2
  zzz1 : Constant  Value=zzz1
  步态函数 : MATLAB Function  TreatAsAtomicUnit=on
  Out1 : Outport
  Out2 : Outport  Port=2
  Out3 : Outport  Port=3
  Out4 : Outport  Port=4
  Out5 : Outport  Port=5
  Out6 : Outport  Port=6
  wires:
  xxx1/1 -> 步态函数/5(xxx1)
  步态函数/17(oz5) -> MuxLeg5/3
  步态函数/7(oy1) -> MuxLeg1/2
  x1/1 -> 步态函数/1(x1)
  x2/1 -> 步态函数/2(x2)
  yyy1/1 -> 步态函数/6(yyy1)
  步态函数/3(ox3) -> MuxLeg3/1
  MuxLeg1/1 -> Out1/1
  zzz1/1 -> 步态函数/8(zzz1)
  步态函数/18(oz6) -> MuxLeg6/3
  步态函数/13(oz1) -> MuxLeg1/3
  MuxLeg4/1 -> Out4/1
  yyy2/1 -> 步态函数/7(yyy2)
  步态函数/16(oz4) -> MuxLeg4/3
  步态函数/2(ox2) -> MuxLeg2/1
  步态函数/5(ox5) -> MuxLeg5/1
  步态函数/10(oy4) -> MuxLeg4/2
  MuxLeg6/1 -> Out6/1
  步态函数/4(ox4) -> MuxLeg4/1
  步态函数/14(oz2) -> MuxLeg2/3
  步态函数/9(oy3) -> MuxLeg3/2
  步态函数/15(oz3) -> MuxLeg3/3
  步态函数/8(oy2) -> MuxLeg2/2
  z2/1 -> 步态函数/4(z2)
  步态函数/11(oy5) -> MuxLeg5/2
  z1/1 -> 步态函数/3(z1)
  步态函数/12(oy6) -> MuxLeg6/2
  步态函数/6(ox6) -> MuxLeg6/1
  步态函数/1(ox1) -> MuxLeg1/1
  MuxLeg2/1 -> Out2/1
  MuxLeg3/1 -> Out3/1
  MuxLeg5/1 -> Out5/1

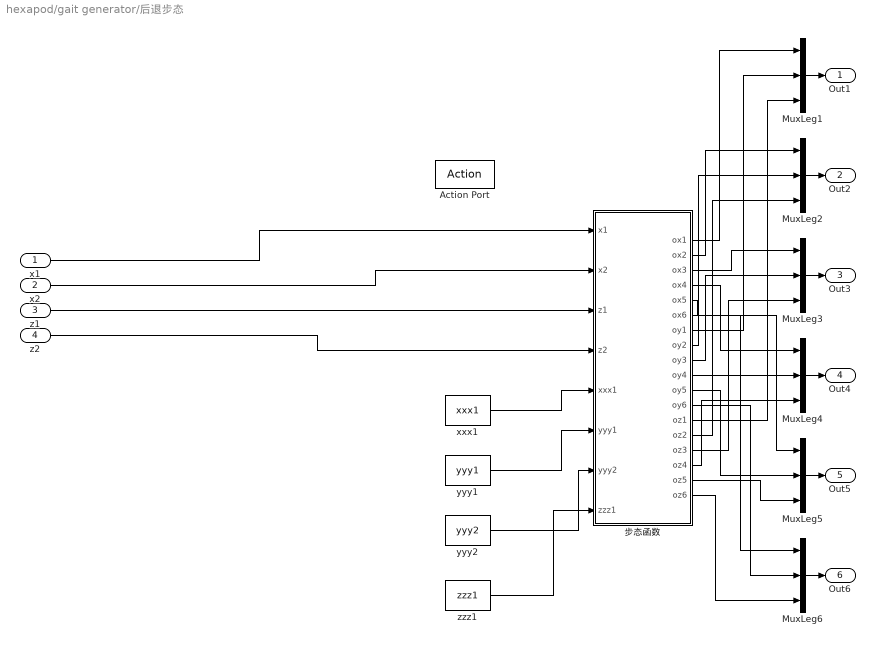
== system hexapod/gait generator/后退步态 ==
  x1 : Inport
  x2 : Inport  Port=2
  z1 : Inport  Port=3
  z2 : Inport  Port=4
  Action Port : ActionPort  ActionPortLabel=elseif(u1==2)
  MuxLeg{1..6} (6 alike) : Mux  Inputs=3
  xxx1 : Constant  Value=xxx1
  yyy1 : Constant  Value=yyy1
  yyy2 : Constant  Value=yyy2
  zzz1 : Constant  Value=zzz1
  步态函数 : MATLAB Function  TreatAsAtomicUnit=on
  Out1 : Outport
  Out2 : Outport  Port=2
  Out3 : Outport  Port=3
  Out4 : Outport  Port=4
  Out5 : Outport  Port=5
  Out6 : Outport  Port=6
  wires:
  xxx1/1 -> 步态函数/5(xxx1)
  步态函数/17(oz5) -> MuxLeg5/3
  步态函数/7(oy1) -> MuxLeg1/2
  x1/1 -> 步态函数/1(x1)
  x2/1 -> 步态函数/2(x2)
  yyy1/1 -> 步态函数/6(yyy1)
  步态函数/3(ox3) -> MuxLeg3/1
  MuxLeg1/1 -> Out1/1
  zzz1/1 -> 步态函数/8(zzz1)
  步态函数/18(oz6) -> MuxLeg6/3
  步态函数/13(oz1) -> MuxLeg1/3
  MuxLeg4/1 -> Out4/1
  yyy2/1 -> 步态函数/7(yyy2)
  步态函数/16(oz4) -> MuxLeg4/3
  步态函数/2(ox2) -> MuxLeg2/1
  步态函数/5(ox5) -> MuxLeg5/1
  步态函数/10(oy4) -> MuxLeg4/2
  MuxLeg6/1 -> Out6/1
  步态函数/4(ox4) -> MuxLeg4/1
  步态函数/14(oz2) -> MuxLeg2/3
  步态函数/9(oy3) -> MuxLeg3/2
  步态函数/15(oz3) -> MuxLeg3/3
  步态函数/8(oy2) -> MuxLeg2/2
  z2/1 -> 步态函数/4(z2)
  步态函数/11(oy5) -> MuxLeg5/2
  z1/1 -> 步态函数/3(z1)
  步态函数/12(oy6) -> MuxLeg6/2
  步态函数/6(ox6) -> MuxLeg6/1
  步态函数/1(ox1) -> MuxLeg1/1
  MuxLeg2/1 -> Out2/1
  MuxLeg3/1 -> Out3/1
  MuxLeg5/1 -> Out5/1

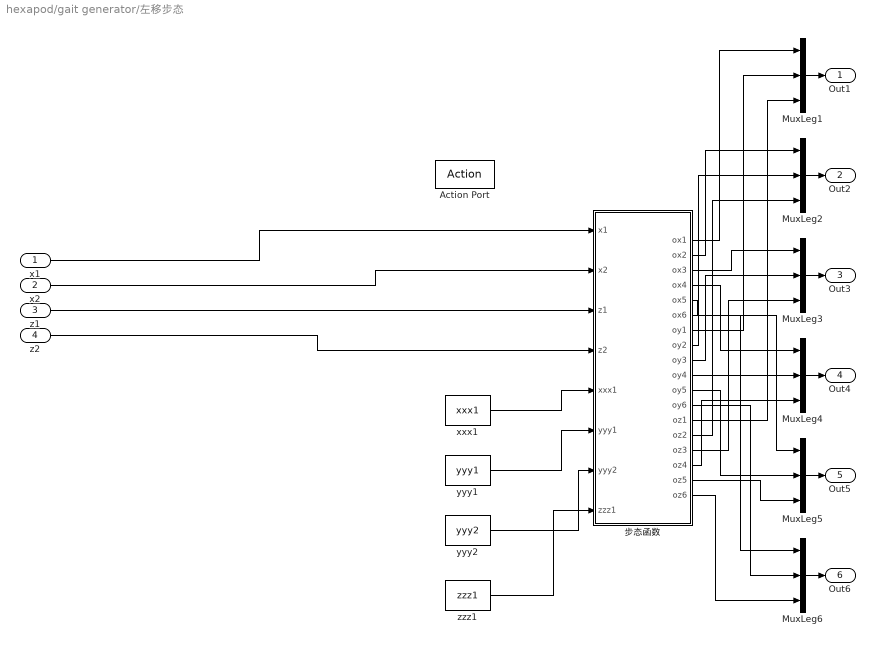
== system hexapod/gait generator/左移步态 ==
  x1 : Inport
  x2 : Inport  Port=2
  z1 : Inport  Port=3
  z2 : Inport  Port=4
  Action Port : ActionPort  ActionPortLabel=elseif(u1==3)
  MuxLeg{1..6} (6 alike) : Mux  Inputs=3
  xxx1 : Constant  Value=xxx1
  yyy1 : Constant  Value=yyy1
  yyy2 : Constant  Value=yyy2
  zzz1 : Constant  Value=zzz1
  步态函数 : MATLAB Function  TreatAsAtomicUnit=on
  Out1 : Outport
  Out2 : Outport  Port=2
  Out3 : Outport  Port=3
  Out4 : Outport  Port=4
  Out5 : Outport  Port=5
  Out6 : Outport  Port=6
  wires:
  MuxLeg5/1 -> Out5/1
  MuxLeg3/1 -> Out3/1
  MuxLeg2/1 -> Out2/1
  步态函数/1(ox1) -> MuxLeg1/1
  步态函数/6(ox6) -> MuxLeg6/1
  步态函数/12(oy6) -> MuxLeg6/2
  z1/1 -> 步态函数/3(z1)
  步态函数/11(oy5) -> MuxLeg5/2
  z2/1 -> 步态函数/4(z2)
  步态函数/8(oy2) -> MuxLeg2/2
  步态函数/15(oz3) -> MuxLeg3/3
  步态函数/9(oy3) -> MuxLeg3/2
  步态函数/14(oz2) -> MuxLeg2/3
  步态函数/4(ox4) -> MuxLeg4/1
  MuxLeg6/1 -> Out6/1
  步态函数/10(oy4) -> MuxLeg4/2
  步态函数/5(ox5) -> MuxLeg5/1
  步态函数/2(ox2) -> MuxLeg2/1
  步态函数/16(oz4) -> MuxLeg4/3
  yyy2/1 -> 步态函数/7(yyy2)
  MuxLeg4/1 -> Out4/1
  步态函数/13(oz1) -> MuxLeg1/3
  步态函数/18(oz6) -> MuxLeg6/3
  zzz1/1 -> 步态函数/8(zzz1)
  MuxLeg1/1 -> Out1/1
  步态函数/3(ox3) -> MuxLeg3/1
  yyy1/1 -> 步态函数/6(yyy1)
  x2/1 -> 步态函数/2(x2)
  x1/1 -> 步态函数/1(x1)
  步态函数/7(oy1) -> MuxLeg1/2
  步态函数/17(oz5) -> MuxLeg5/3
  xxx1/1 -> 步态函数/5(xxx1)

== system hexapod/gait generator/足尖轨迹生成 ==
  H : Constant  Value=H
  L : Constant  Value=L
  Repeating Sequence : simulink/Sources/Repeating Sequence  rep_seq_t=[0 1]  rep_seq_y=[0 1]
  Scope1 : Scope  NumInputPorts=4
  Transport Delay : TransportDelay  DelayTime=0.5
  Transport Delay1 : TransportDelay  DelayTime=0.5
  x : MATLAB Function  TreatAsAtomicUnit=on
  z : MATLAB Function  TreatAsAtomicUnit=on
  x1 : Outport
  x2 : Outport  Port=2
  z1 : Outport  Port=3
  z2 : Outport  Port=4
  LL : Outport  Port=5
  wires:
  x/1(x) -> Transport Delay/1, x1/1, Scope1/1
  Transport Delay1/1 -> z2/1, Scope1/4
  Transport Delay/1 -> x2/1, Scope1/2
  z/1(z) -> Transport Delay1/1, z1/1, Scope1/3
  H/1 -> z/2(H)
  Repeating Sequence/1 -> z/1(t), x/1(t)
  L/1 -> x/2(L), LL/1

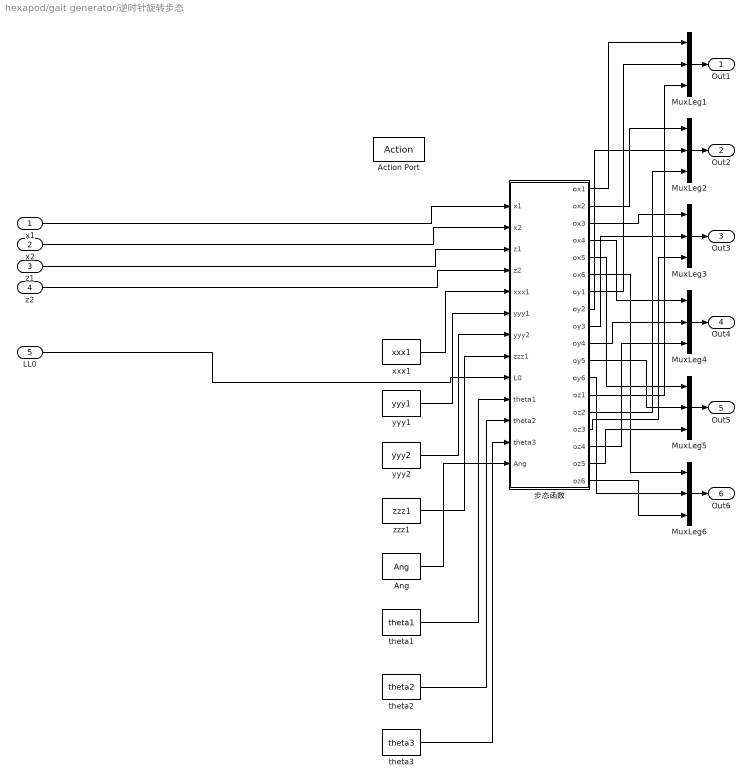
== system hexapod/gait generator/逆时针旋转步态 ==
  x1 : Inport
  x2 : Inport  Port=2
  z1 : Inport  Port=3
  z2 : Inport  Port=4
  LL0 : Inport  Port=5
  Action Port : ActionPort  ActionPortLabel=elseif(u1==6)
  Ang : Constant  Value=Ang
  MuxLeg{1..6} (6 alike) : Mux  Inputs=3
  theta1 : Constant  Value=theta1
  theta2 : Constant  Value=theta2
  theta3 : Constant  Value=theta3
  xxx1 : Constant  Value=xxx1
  yyy1 : Constant  Value=yyy1
  yyy2 : Constant  Value=yyy2
  zzz1 : Constant  Value=zzz1
  步态函数 : MATLAB Function  TreatAsAtomicUnit=on
  Out1 : Outport
  Out2 : Outport  Port=2
  Out3 : Outport  Port=3
  Out4 : Outport  Port=4
  Out5 : Outport  Port=5
  Out6 : Outport  Port=6
  wires:
  xxx1/1 -> 步态函数/5(xxx1)
  步态函数/17(oz5) -> MuxLeg5/3
  步态函数/7(oy1) -> MuxLeg1/2
  x1/1 -> 步态函数/1(x1)
  x2/1 -> 步态函数/2(x2)
  yyy1/1 -> 步态函数/6(yyy1)
  步态函数/3(ox3) -> MuxLeg3/1
  MuxLeg1/1 -> Out1/1
  zzz1/1 -> 步态函数/8(zzz1)
  步态函数/18(oz6) -> MuxLeg6/3
  步态函数/13(oz1) -> MuxLeg1/3
  MuxLeg4/1 -> Out4/1
  yyy2/1 -> 步态函数/7(yyy2)
  步态函数/16(oz4) -> MuxLeg4/3
  步态函数/2(ox2) -> MuxLeg2/1
  步态函数/5(ox5) -> MuxLeg5/1
  步态函数/10(oy4) -> MuxLeg4/2
  MuxLeg6/1 -> Out6/1
  步态函数/4(ox4) -> MuxLeg4/1
  步态函数/14(oz2) -> MuxLeg2/3
  步态函数/9(oy3) -> MuxLeg3/2
  步态函数/15(oz3) -> MuxLeg3/3
  步态函数/8(oy2) -> MuxLeg2/2
  z2/1 -> 步态函数/4(z2)
  步态函数/11(oy5) -> MuxLeg5/2
  z1/1 -> 步态函数/3(z1)
  步态函数/12(oy6) -> MuxLeg6/2
  步态函数/6(ox6) -> MuxLeg6/1
  步态函数/1(ox1) -> MuxLeg1/1
  MuxLeg2/1 -> Out2/1
  MuxLeg3/1 -> Out3/1
  MuxLeg5/1 -> Out5/1
  LL0/1 -> 步态函数/9(L0)
  theta1/1 -> 步态函数/10(theta1)
  theta2/1 -> 步态函数/11(theta2)
  theta3/1 -> 步态函数/12(theta3)
  Ang/1 -> 步态函数/13(Ang)

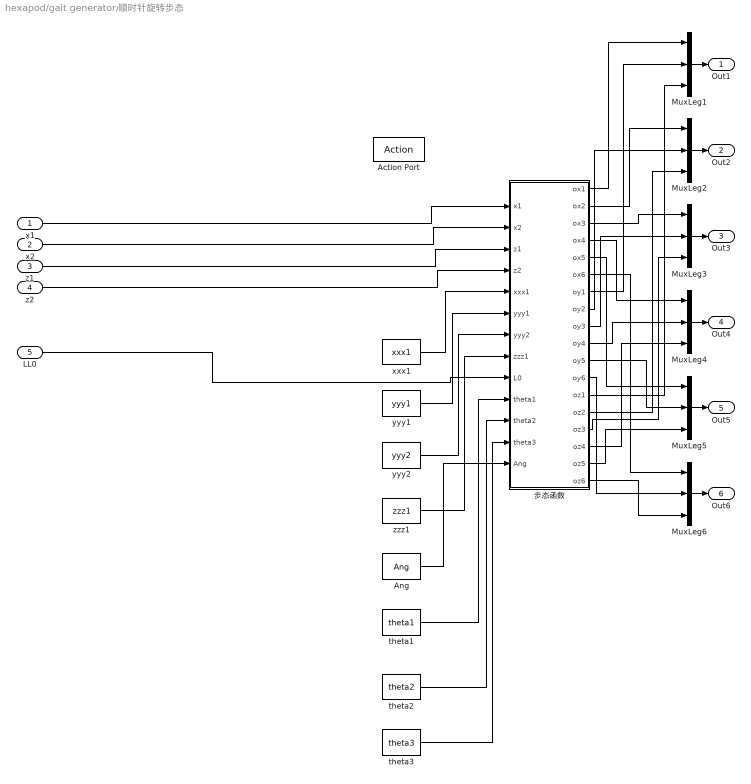
== system hexapod/gait generator/顺时针旋转步态 ==
  x1 : Inport
  x2 : Inport  Port=2
  z1 : Inport  Port=3
  z2 : Inport  Port=4
  LL0 : Inport  Port=5
  Action Port : ActionPort  ActionPortLabel=elseif(u1==5)
  Ang : Constant  Value=Ang
  MuxLeg{1..6} (6 alike) : Mux  Inputs=3
  theta1 : Constant  Value=theta1
  theta2 : Constant  Value=theta2
  theta3 : Constant  Value=theta3
  xxx1 : Constant  Value=xxx1
  yyy1 : Constant  Value=yyy1
  yyy2 : Constant  Value=yyy2
  zzz1 : Constant  Value=zzz1
  步态函数 : MATLAB Function  TreatAsAtomicUnit=on
  Out1 : Outport
  Out2 : Outport  Port=2
  Out3 : Outport  Port=3
  Out4 : Outport  Port=4
  Out5 : Outport  Port=5
  Out6 : Outport  Port=6
  wires:
  Ang/1 -> 步态函数/13(Ang)
  theta3/1 -> 步态函数/12(theta3)
  theta2/1 -> 步态函数/11(theta2)
  theta1/1 -> 步态函数/10(theta1)
  LL0/1 -> 步态函数/9(L0)
  MuxLeg5/1 -> Out5/1
  MuxLeg3/1 -> Out3/1
  MuxLeg2/1 -> Out2/1
  步态函数/1(ox1) -> MuxLeg1/1
  步态函数/6(ox6) -> MuxLeg6/1
  步态函数/12(oy6) -> MuxLeg6/2
  z1/1 -> 步态函数/3(z1)
  步态函数/11(oy5) -> MuxLeg5/2
  z2/1 -> 步态函数/4(z2)
  步态函数/8(oy2) -> MuxLeg2/2
  步态函数/15(oz3) -> MuxLeg3/3
  步态函数/9(oy3) -> MuxLeg3/2
  步态函数/14(oz2) -> MuxLeg2/3
  步态函数/4(ox4) -> MuxLeg4/1
  MuxLeg6/1 -> Out6/1
  步态函数/10(oy4) -> MuxLeg4/2
  步态函数/5(ox5) -> MuxLeg5/1
  步态函数/2(ox2) -> MuxLeg2/1
  步态函数/16(oz4) -> MuxLeg4/3
  yyy2/1 -> 步态函数/7(yyy2)
  MuxLeg4/1 -> Out4/1
  步态函数/13(oz1) -> MuxLeg1/3
  步态函数/18(oz6) -> MuxLeg6/3
  zzz1/1 -> 步态函数/8(zzz1)
  MuxLeg1/1 -> Out1/1
  步态函数/3(ox3) -> MuxLeg3/1
  yyy1/1 -> 步态函数/6(yyy1)
  x2/1 -> 步态函数/2(x2)
  x1/1 -> 步态函数/1(x1)
  步态函数/7(oy1) -> MuxLeg1/2
  步态函数/17(oz5) -> MuxLeg5/3
  xxx1/1 -> 步态函数/5(xxx1)

== system hexapod/Leg1/leg1/link1 ==
  Cylindrical Solid1 : sm_lib/Body Elements/Cylindrical Solid  GraphicAmbientColor=[0.15 0.15 0.15 1.0]  BasedOnType=Density  CenterOfMass=[0 0 0]  CenterOfMassUnits=m  GraphicDiffuseColor=[0.5 0.5 0.5]  CylinderLength=45  CylinderLengthUnits=mm  CylinderRadius=12.5  CylinderRadiusUnits=mm  Density=1000  DensityUnits=kg/m^3  DoExposeReferenceFrame=on  GraphicEmissiveColor=[0.0 0.0 0.0 1.0]  ExportEntireGeometry=off  SerializedFrames=<Frames/>  MarkerShape=Sphere  MarkerSize=10  GraphicType=FromGeometry  InertiaType=CalculateFromGeometry  Mass=1  MassUnits=kg  MomentsOfInertia=[1 1 1]  MomentsOfInertiaUnits=kg*m^2  GraphicOpacity=1.0  ProductsOfInertia=[0 0 0]  ProductsOfInertiaUnits=kg*m^2  GraphicShininess=75  GraphicSpecularColor=[0.5 0.5 0.5 1.0]  GraphicVisPropType=SimpleVisualProperties
  O1_j1a : sm_lib/Frames and Transforms/Rigid Transform  TranslationMethod=Cartesian  TranslationStandardOffset=0  TranslationLengthUnit=mm  TranslationStandardAxis=+Z  TranslationCartesianOffset=[45 0 0]  TranslationROffset=0  TranslationROffsetUnits=m  TranslationZOffset=0  TranslationZOffsetUnits=m  TranslationThetaOffset=0  TranslationThetaOffsetUnits=deg  RotationMethod=StandardAxis  RotationAngleUnits=deg  RotationStandardAxis=+X  RotationAngle=90  RotationArbitraryAxis=[0 0 1]  FollAlignAxisA=+X  BaseAlignAxisA=+Y  FollAlignAxisB=+Y  BaseAlignAxisB=+Z  RotationSequenceAxes=FollowerAxes  RotationSequence=XYX  RotationSequenceAngles=[0 0 0]  RotationSequenceAnglesUnits=deg  RotationMatrix=[1 0 0; 0 1 0; 0 0 1]
  O1_j1b : sm_lib/Frames and Transforms/Rigid Transform  TranslationMethod=None  TranslationStandardOffset=0  TranslationLengthUnit=mm  TranslationStandardAxis=+Z  TranslationCartesianOffset=[45 0 0]  TranslationROffset=0  TranslationROffsetUnits=m  TranslationZOffset=0  TranslationZOffsetUnits=m  TranslationThetaOffset=0  TranslationThetaOffsetUnits=deg  RotationMethod=StandardAxis  RotationAngleUnits=deg  RotationStandardAxis=+Z  RotationAngle=90  RotationArbitraryAxis=[0 0 1]  FollAlignAxisA=+X  BaseAlignAxisA=+Y  FollAlignAxisB=+Y  BaseAlignAxisB=+Z  RotationSequenceAxes=FollowerAxes  RotationSequence=XYX  RotationSequenceAngles=[0 0 0]  RotationSequenceAnglesUnits=deg  RotationMatrix=[1 0 0; 0 1 0; 0 0 1]
  bias_j1i1 : sm_lib/Frames and Transforms/Rigid Transform  TranslationMethod=Cartesian  TranslationStandardOffset=0  TranslationLengthUnit=mm  TranslationStandardAxis=+Z  TranslationCartesianOffset=[45/2 0 0]  TranslationROffset=0  TranslationROffsetUnits=m  TranslationZOffset=0  TranslationZOffsetUnits=m  TranslationThetaOffset=0  TranslationThetaOffsetUnits=deg  RotationMethod=StandardAxis  RotationAngleUnits=deg  RotationStandardAxis=+Y  RotationAngle=90  RotationArbitraryAxis=[0 0 1]  FollAlignAxisA=+X  BaseAlignAxisA=+Y  FollAlignAxisB=+Y  BaseAlignAxisB=+Z  RotationSequenceAxes=FollowerAxes  RotationSequence=XYX  RotationSequenceAngles=[0 0 0]  RotationSequenceAnglesUnits=deg  RotationMatrix=[1 0 0; 0 1 0; 0 0 1]
  Conn1 : PMIOPort  Side=Left
  Conn2 : PMIOPort  Port=2  Side=Right
  connections:
  O1_j1b/RConn1 -- Conn2/RConn1
  O1_j1b/LConn1 -- O1_j1a/RConn1
  bias_j1i1/RConn1 -- Cylindrical Solid1/RConn1
  bias_j1i1/LConn1 -- Conn1/RConn1 -- O1_j1a/LConn1

== system hexapod/Leg1/leg1/link2 ==
  O2_j2 : sm_lib/Frames and Transforms/Rigid Transform  TranslationMethod=Cartesian  TranslationStandardOffset=0  TranslationLengthUnit=mm  TranslationStandardAxis=+Z  TranslationCartesianOffset=[93.5 0 0]  TranslationROffset=0  TranslationROffsetUnits=m  TranslationZOffset=0  TranslationZOffsetUnits=m  TranslationThetaOffset=0  TranslationThetaOffsetUnits=deg  RotationMethod=StandardAxis  RotationAngleUnits=deg  RotationStandardAxis=-Z  RotationAngle=169.09  RotationArbitraryAxis=[0 0 1]  FollAlignAxisA=+X  BaseAlignAxisA=+Y  FollAlignAxisB=+Y  BaseAlignAxisB=+Z  RotationSequenceAxes=FollowerAxes  RotationSequence=XYX  RotationSequenceAngles=[0 0 0]  RotationSequenceAnglesUnits=deg  RotationMatrix=[1 0 0; 0 1 0; 0 0 1]
  bias_j2 : sm_lib/Frames and Transforms/Rigid Transform  TranslationMethod=Cartesian  TranslationStandardOffset=0  TranslationLengthUnit=mm  TranslationStandardAxis=+Z  TranslationCartesianOffset=[93.5/2 0 0]  TranslationROffset=0  TranslationROffsetUnits=m  TranslationZOffset=0  TranslationZOffsetUnits=m  TranslationThetaOffset=0  TranslationThetaOffsetUnits=deg  RotationMethod=StandardAxis  RotationAngleUnits=deg  RotationStandardAxis=+Y  RotationAngle=90  RotationArbitraryAxis=[0 0 1]  FollAlignAxisA=+X  BaseAlignAxisA=+Y  FollAlignAxisB=+Y  BaseAlignAxisB=+Z  RotationSequenceAxes=FollowerAxes  RotationSequence=XYX  RotationSequenceAngles=[0 0 0]  RotationSequenceAnglesUnits=deg  RotationMatrix=[1 0 0; 0 1 0; 0 0 1]
  leg2 : sm_lib/Body Elements/Cylindrical Solid  GraphicAmbientColor=[0.15 0.15 0.15 1.0]  BasedOnType=Density  CenterOfMass=[0 0 0]  CenterOfMassUnits=m  GraphicDiffuseColor=[0.5 0.5 0.5]  CylinderLength=93.5  CylinderLengthUnits=mm  CylinderRadius=12.5  CylinderRadiusUnits=mm  Density=1000  DensityUnits=kg/m^3  DoExposeReferenceFrame=on  GraphicEmissiveColor=[0.0 0.0 0.0 1.0]  ExportEntireGeometry=off  SerializedFrames=<Frames/>  MarkerShape=Sphere  MarkerSize=10  GraphicType=FromGeometry  InertiaType=CalculateFromGeometry  Mass=1  MassUnits=kg  MomentsOfInertia=[1 1 1]  MomentsOfInertiaUnits=kg*m^2  GraphicOpacity=1.0  ProductsOfInertia=[0 0 0]  ProductsOfInertiaUnits=kg*m^2  GraphicShininess=75  GraphicSpecularColor=[0.5 0.5 0.5 1.0]  GraphicVisPropType=SimpleVisualProperties
  Conn1 : PMIOPort  Side=Left
  Conn2 : PMIOPort  Port=2  Side=Right
  connections:
  Conn1/RConn1 -- bias_j2/LConn1 -- O2_j2/LConn1
  O2_j2/RConn1 -- Conn2/RConn1
  bias_j2/RConn1 -- leg2/RConn1
